simulink model "open_loop"  (R2023b)
settings: Solver=VariableStepAuto  StartTime=0.0  StopTime=10.0  RelTol=1e-3
undefined symbols (not defined in the file or in its folder): a_m, config, K_g, K_m
settings Model: Creator=foderking  LastModifiedBy=foderking

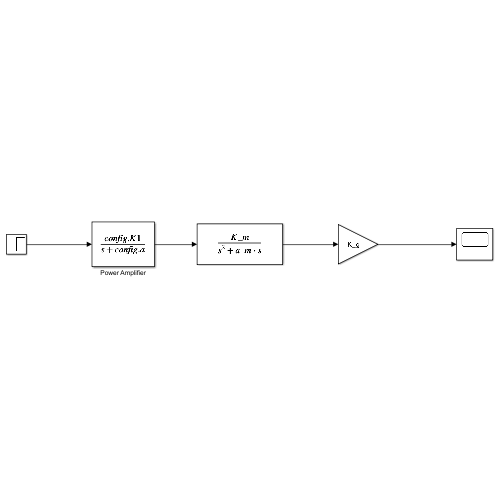
[thumbnail: Simulink's stored preview of the top-level diagram]
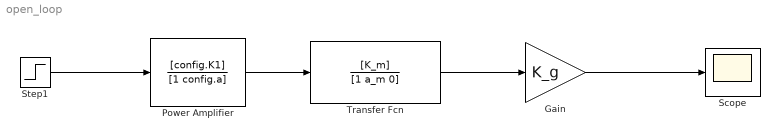
== system open_loop ==
  Gain : Gain  Gain=K_g
  Power Amplifier : TransferFcn  Numerator=[config.K1]  Denominator=[1 config.a]
  Scope : Scope
  Step1 : Step  SampleTime=0
  Transfer Fcn : TransferFcn  Numerator=[K_m]  Denominator=[1 a_m 0]
  wires:
  Power Amplifier/1 -> Transfer Fcn/1
  Transfer Fcn/1 -> Gain/1
  Gain/1 -> Scope/1
  Step1/1 -> Power Amplifier/1
